simulink model "Carrito"  (R2013a)
settings: Solver=ode45  StartTime=0.0  StopTime=10.0  RelTol=1e-3
InitFcn:
  | M=0.2;m=0.1;l=0.3;B1=0.1;B2=0.1;g=9.81;
settings Model: Creator=LuisFernando  LastModifiedBy=LuisFernando

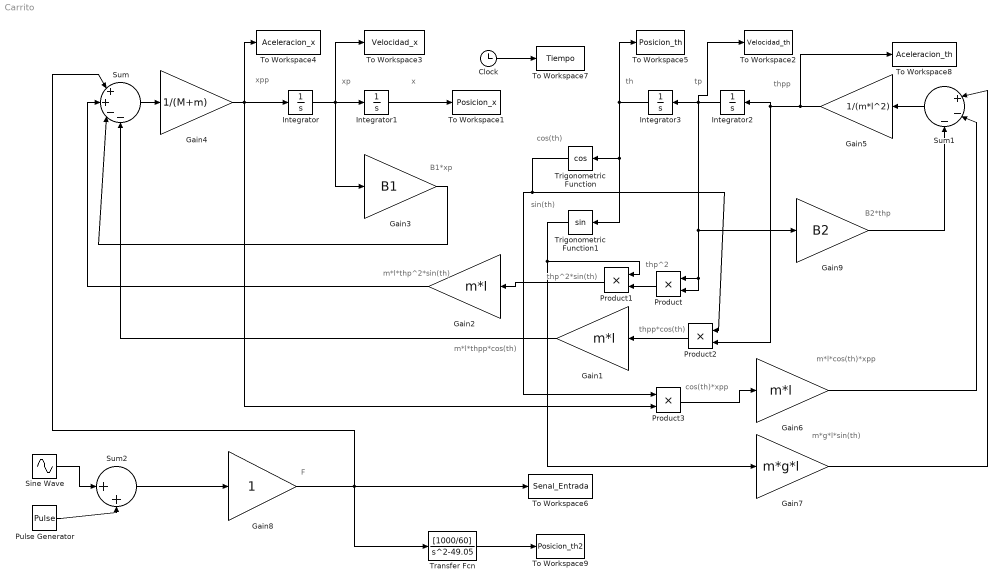
== system Carrito ==
  note: B1*xp
  note: B2*thp
  note: m*g*l*sin(th)
  note: m*l*cos(th)*xpp
  note: cos(th)*xpp
  note: m*l*thpp*cos(th)
  note: m*l*thp^2*sin(th)
  note: thpp*cos(th)
  note: thp^2*sin(th)
  note: thp^2
  note: sin(th)
  note: cos(th)
  note: xpp
  note: x
  note: xp
  note: thpp
  note: th
  note: tp
  note: F
  Clock : Clock
      settings: Decimation=100
  Gain1 : Gain  Gain=m*l
  Gain2 : Gain  Gain=m*l
  Gain3 : Gain  Gain=B1
  Gain4 : Gain  Gain=1/(M+m)
  Gain5 : Gain  Gain=1/(m*l^2)
  Gain6 : Gain  Gain=m*l
  Gain7 : Gain  Gain=m*g*l
  Gain8 : Gain
  Gain9 : Gain  Gain=B2
  Integrator : Integrator
  Integrator1 : Integrator
  Integrator2 : Integrator
  Integrator3 : Integrator  InitialCondition=pi/2  LimitOutput=on  UpperSaturationLimit=pi  LowerSaturationLimit=-pi
  Product{,1..3} (4 alike) : Product
  Pulse Generator : DiscretePulseGenerator  PulseType=Time based  Amplitude=0.1  Period=1  PulseWidth=50
  Sine Wave : Sin  Amplitude=0  SampleTime=0
  Sum : Sum  Inputs=|++--
  Sum1 : Sum  Inputs=|+--
  Sum2 : Sum  Inputs=|++
  To Workspace1 : ToWorkspace  VariableName=Posicion_x  SampleTime=0.01
  To Workspace2 : ToWorkspace  VariableName=Velocidad_th  SampleTime=0.01
  To Workspace3 : ToWorkspace  VariableName=Velocidad_x  SampleTime=0.01
  To Workspace4 : ToWorkspace  VariableName=Aceleracion_x  SampleTime=0.01
  To Workspace5 : ToWorkspace  VariableName=Posicion_th  SampleTime=0.01
  To Workspace6 : ToWorkspace  VariableName=Senal_Entrada  SampleTime=0.01
  To Workspace7 : ToWorkspace  VariableName=Tiempo  SampleTime=0.01
  To Workspace8 : ToWorkspace  VariableName=Aceleracion_th  SampleTime=0.01
  To Workspace9 : ToWorkspace  VariableName=Posicion_th2  SampleTime=0.01
  Transfer Fcn : TransferFcn  Numerator=[1000/60]  Denominator=[1 0 -49.05]
  Trigonometric Function : Trigonometry  Operator=cos
  Trigonometric Function1 : Trigonometry
  wires:
  Integrator/1 -> Gain3/1, Integrator1/1, To Workspace3/1
  Integrator3/1 -> Trigonometric Function1/1, Trigonometric Function/1, To Workspace5/1
  Integrator2/1 -> Gain9/1, Product/2, Product/1, Integrator3/1, To Workspace2/1
  Integrator1/1 -> To Workspace1/1
  Clock/1 -> To Workspace7/1
  Sine Wave/1 -> Sum2/1
  Pulse Generator/1 -> Sum2/2
  Sum2/1 -> Gain8/1
  Gain8/1 -> Transfer Fcn/1, To Workspace6/1, Sum/1
  Trigonometric Function1/1 -> Gain7/1, Product1/1
  Product/1 -> Product1/2
  Product1/1 -> Gain2/1
  Product2/1 -> Gain1/1
  Trigonometric Function/1 -> Product3/1, Product2/1
  Gain4/1 -> Product3/2, Integrator/1, To Workspace4/1
  Sum/1 -> Gain4/1
  Gain3/1 -> Sum/3
  Gain1/1 -> Sum/4
  Gain2/1 -> Sum/2
  Gain5/1 -> To Workspace8/1, Integrator2/1, Product2/2
  Sum1/1 -> Gain5/1
  Product3/1 -> Gain6/1
  Gain9/1 -> Sum1/3
  Gain6/1 -> Sum1/2
  Gain7/1 -> Sum1/1
  Transfer Fcn/1 -> To Workspace9/1
